simulink library "INP_IMU_Prep"  (R2023b)
settings: Solver=VariableStepAuto  StartTime=0.0  StopTime=10.0  RelTol=1e-3
undefined symbols (not defined in the file): INP_IMU_c_TiSample_s, INP_IMU_p_AVehLgtOfs_mps2, INP_IMU_p_AVehLgtSca_na, INP_IMU_p_TauFilt_s
libraries: VUT_lib x3
settings Model: Creator=blatak  LastModifiedBy=blatak
settings ModelReferenceCC: EnableRefExpFcnMdlSchedulingChecks=on

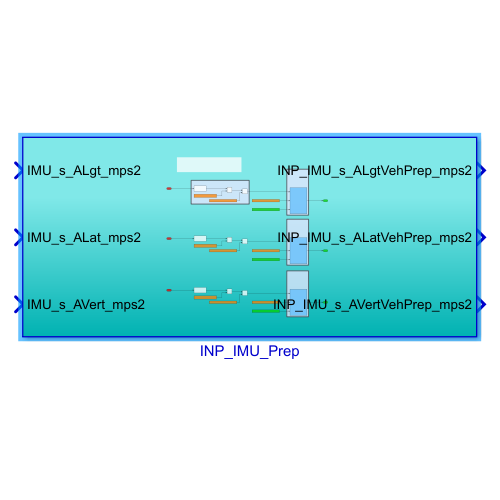
[thumbnail: Simulink's stored preview of the top-level diagram]
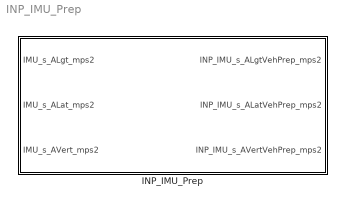
== system INP_IMU_Prep ==
  INP_IMU_Prep : Subsystem

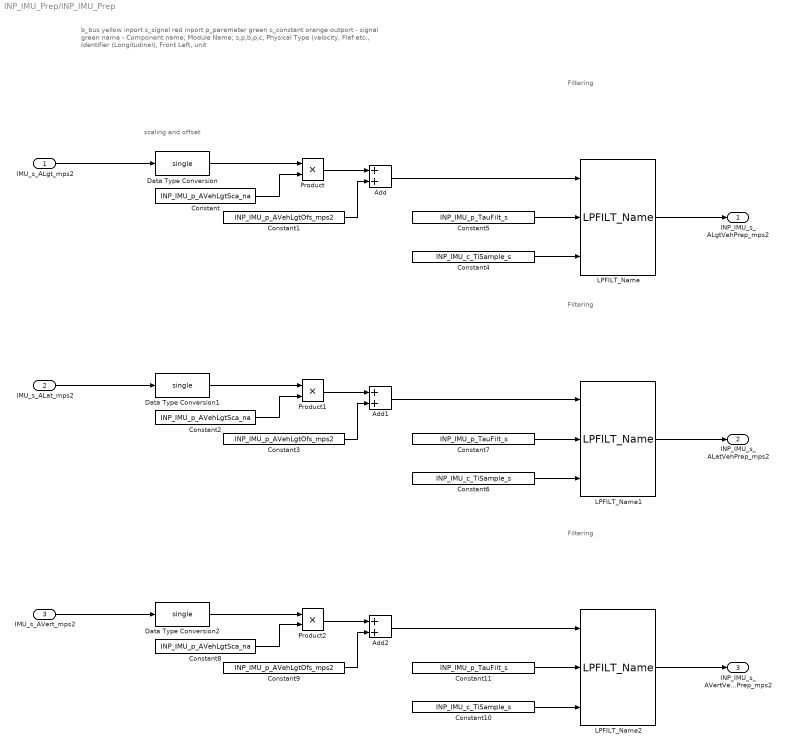
== system INP_IMU_Prep/INP_IMU_Prep ==
  note: Filtering
  note: b_bus yellow inport
      | s_signal red inport
      | p_parameter green
      | c_constant orange
      | outport - signal green
      | name - Component name; Module Name; s,p,b,p,c, Physical Type (velocity, Flaf etc., Identifier (Longitudinal), Front Left, unit
  note: scaling and offset
  note: Filtering
  note: Filtering
  IMU_s_ALgt_mps2 : Inport
  IMU_s_ALat_mps2 : Inport  Port=2
  IMU_s_AVert_mps2 : Inport  Port=3
  Add : Sum
  Add1 : Sum
  Add2 : Sum
  Constant : Constant  Value=INP_IMU_p_AVehLgtSca_na
  Constant1 : Constant  Value=INP_IMU_p_AVehLgtOfs_mps2
  Constant10 : Constant  Value=INP_IMU_c_TiSample_s
  Constant11 : Constant  Value=INP_IMU_p_TauFilt_s
  Constant2 : Constant  Value=INP_IMU_p_AVehLgtSca_na
  Constant3 : Constant  Value=INP_IMU_p_AVehLgtOfs_mps2
  Constant4 : Constant  Value=INP_IMU_c_TiSample_s
  Constant5 : Constant  Value=INP_IMU_p_TauFilt_s
  Constant6 : Constant  Value=INP_IMU_c_TiSample_s
  Constant7 : Constant  Value=INP_IMU_p_TauFilt_s
  Constant8 : Constant  Value=INP_IMU_p_AVehLgtSca_na
  Constant9 : Constant  Value=INP_IMU_p_AVehLgtOfs_mps2
  Data Type Conversion : DataTypeConversion  OutDataTypeStr=single  SaturateOnIntegerOverflow=off  RndMeth=Floor
  Data Type Conversion1 : DataTypeConversion  OutDataTypeStr=single  SaturateOnIntegerOverflow=off  RndMeth=Floor
  Data Type Conversion2 : DataTypeConversion  OutDataTypeStr=single  SaturateOnIntegerOverflow=off  RndMeth=Floor
  LPFILT_Name : VUT_lib/LPFILT_Name  SystemSampleTime=-1  VariantActivationTime=update diagram  AllowFlexibleInterface=on  Latency=0  AutoFrameSizeCalculation=off
  LPFILT_Name1 : VUT_lib/LPFILT_Name  SystemSampleTime=-1  VariantActivationTime=update diagram  AllowFlexibleInterface=on  Latency=0  AutoFrameSizeCalculation=off
  LPFILT_Name2 : VUT_lib/LPFILT_Name  SystemSampleTime=-1  VariantActivationTime=update diagram  AllowFlexibleInterface=on  Latency=0  AutoFrameSizeCalculation=off
  Product : Product
  Product1 : Product
  Product2 : Product
  INP_IMU_s_ALgtVehPrep_mps2 : Outport
  INP_IMU_s_ALatVehPrep_mps2 : Outport  Port=2
  INP_IMU_s_AVertVehPrep_mps2 : Outport  Port=3
  wires:
  Data Type Conversion/1 -> Product/1
  Product/1 -> Add/1
  Constant1/1 -> Add/2
  Constant/1 -> Product/2
  IMU_s_ALgt_mps2/1 -> Data Type Conversion/1
  LPFILT_Name/1 -> INP_IMU_s_ALgtVehPrep_mps2/1
  Add/1 -> LPFILT_Name/1
  Constant3/1 -> Add1/2
  Product1/1 -> Add1/1
  Constant2/1 -> Product1/2
  Data Type Conversion1/1 -> Product1/1
  IMU_s_ALat_mps2/1 -> Data Type Conversion1/1
  Constant4/1 -> LPFILT_Name/3
  Constant5/1 -> LPFILT_Name/2
  Constant6/1 -> LPFILT_Name1/3
  Constant7/1 -> LPFILT_Name1/2
  Add1/1 -> LPFILT_Name1/1
  Constant10/1 -> LPFILT_Name2/3
  Constant9/1 -> Add2/2
  Constant11/1 -> LPFILT_Name2/2
  Product2/1 -> Add2/1
  Constant8/1 -> Product2/2
  IMU_s_AVert_mps2/1 -> Data Type Conversion2/1
  Data Type Conversion2/1 -> Product2/1
  Add2/1 -> LPFILT_Name2/1
  LPFILT_Name1/1 -> INP_IMU_s_ALatVehPrep_mps2/1
  LPFILT_Name2/1 -> INP_IMU_s_AVertVehPrep_mps2/1
